simulink library "inp"  (R2021b)
settings: Solver=VariableStepAuto  StartTime=0.0  StopTime=10.0  RelTol=1e-3
undefined symbols (not defined in the file): C_TASK_5MS_S, FALSE, KINP_AcoreReadyToSlp_flg_ovrdflg, KINP_AcoreReadyToSlp_flg_ovrdval, KINP_AllowMovThd_OTA_enum_ovrdflg, KINP_AllowMovThd_OTA_enum_ovrdval, KINP_APSAngleTarget_Deg_ovrdflg, KINP_APSAngleTarget_Deg_ovrdval, KINP_APSDecReq_mps2_ovrdflg, KINP_APSDecReq_mps2_ovrdval, KINP_APSDecReqA_flg_ovrdflg, KINP_APSDecReqA_flg_ovrdval, KINP_APSDFLL_cm_ovrdflg, KINP_APSDFLL_cm_ovrdval, KINP_APSDFLR_cm_ovrdflg, KINP_APSDFLR_cm_ovrdval, KINP_APSDRLL_cm_ovrdflg, KINP_APSDRLL_cm_ovrdval, KINP_APSDRLR_cm_ovrdflg, KINP_APSDRLR_cm_ovrdval, KINP_APSExitCondition_enum_ovrdflg, KINP_APSExitCondition_enum_ovrdval, KINP_APSHWVer_enum_ovrdflg, KINP_APSHWVer_enum_ovrdval, KINP_APSProgressPCT_pct_ovrdflg, KINP_APSProgressPCT_pct_ovrdval, KINP_APSReq_enum_ovrdflg, KINP_APSReq_enum_ovrdval, KINP_APSRQDisplay_enum_ovrdflg, KINP_APSRQDisplay_enum_ovrdval, KINP_APSRqEPASCtrl_flg_ovrdflg, KINP_APSRqEPASCtrl_flg_ovrdval, KINP_APSShiftPosnReq_enum_ovrdval, KINP_APSShiftPosnReq_enum_ovrflg, KINP_APSSpeedCMD_kph_ovrdval, KINP_APSSpeedCMD_kph_ovrflg, KINP_APSStaSystem_enum_ovrdflg, KINP_APSStaSystem_enum_ovrdval, KINP_APSSWVer_enum_ovrdflg, KINP_APSSWVer_enum_ovrdval, KINP_APSVMCReqA_flg_ovrdval, KINP_APSVMCReqA_flg_ovrflg, KINP_APSVRqEPASCtrl_flg_ovrdflg, KINP_APSVRqEPASCtrl_flg_ovrdval, KINP_AuxBattVolmV_mV_ovrdflg, KINP_AuxBattVolmV_mV_ovrdval, KINP_CAASSta_enum_ovrdflg, KINP_CAASSta_enum_ovrdval, KINP_CAASVMCReqA_flg_ovrdval, KINP_CAASVMCReqA_flg_ovrflg, KINP_Chime_enum_ovrdflg, KINP_Chime_enum_ovrdval, KINP_ClearDTCcmd_flg_ovrdflg, KINP_ClearDTCcmd_flg_ovrdval, KINP_EvccAplusPwrUpReq_flg_ovrdflg, KINP_EvccAplusPwrUpReq_flg_ovrdval, KINP_LFID_raw_ovrdval, KINP_LFID_raw_ovrflg, KINP_LRID_raw_ovrdval, KINP_MemOffsetAccX_raw16_ovrdflg ... (+118)
libraries: FVT_lib x942, hcu_lib x1
(part 9 of 31)

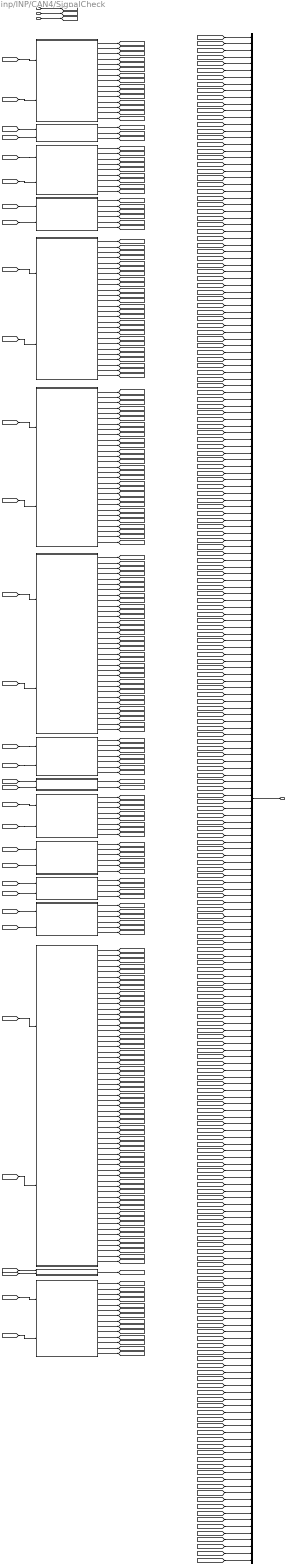
== system inp/INP/CAN4/SignalCheck ==
  inp_CanValid_bus : Inport
  TASK_TIME_S : Inport  Port=2
  BHAL_outputs : Inport  Port=3
  DKC1 : Subsystem
  DKC2 : Subsystem
  PTG1 : Subsystem
  ZONE_DR1 : Subsystem
  ZONE_DR_VCU : Subsystem
  ZONE_FR1 : Subsystem
  ZONE_FR_VCU : Subsystem
  ZONE_L1 : Subsystem
  ZONE_L2 : Subsystem
  ZONE_R1 : Subsystem
  ZONE_R2 : Subsystem
  bus_creator : BusCreator  Inputs=228
  zGW_APTC1 : Subsystem
  zGW_CANFr1 : Subsystem
  zGW_LINDr1 : Subsystem
  zGW_LINFr1 : Subsystem
  zGW_SEAT1 : Subsystem
  inp_Hal_bus : Outport
  wires:
  inp_CanValid_bus/1 -> [inp_CanValid_bus]
  TASK_TIME_S/1 -> [TASK_TIME_S]
  BHAL_outputs/1 -> [BHAL_outputs]
  [BHAL_outputs] -> DKC1/1(BHAL_outputs)
  [inp_CanValid_bus] -> DKC1/2(inp_CanValid_bus)
  DKC1/1(VINP_DKCKeyNumSta_enum) -> [VINP_DKCKeyNumSta_enum]
  DKC1/2(VINP_DKCKeyTypeSta_enum) -> [VINP_DKCKeyTypeSta_enum]
  DKC1/3(VINP_DKCPDkeyAreaRAPSSta_enum) -> [VINP_DKCPDkeyAreaRAPSSta_enum]
  DKC1/4(VINP_DKCParkingModeCmd_enum) -> [VINP_DKCParkingModeCmd_enum]
  DKC1/5(VINP_DKCReVehData_enum) -> [VINP_DKCReVehData_enum]
  DKC1/6(VINP_PCommandToBCM_enum) -> [VINP_PCommandToBCM_enum]
  DKC1/7(VINP_PCommandToPTG_enum) -> [VINP_PCommandToPTG_enum]
  DKC1/8(VINP_PDKeyAreaLockUnlock_enum) -> [VINP_PDKeyAreaLockUnlock_enum]
  DKC1/9(VINP_PDKeyAreaPS_enum) -> [VINP_PDKeyAreaPS_enum]
  DKC1/10(VINP_PDKeyAreaPTG_enum) -> [VINP_PDKeyAreaPTG_enum]
  DKC1/11(VINP_PDKeyWelcome_enum) -> [VINP_PDKeyWelcome_enum]
  DKC1/12(VINP_PDkeyShowIVI_enum) -> [VINP_PDkeyShowIVI_enum]
  DKC1/13(VINP_PKeyMiss_flg) -> [VINP_PKeyMiss_flg]
  DKC1/14(VINP_PKeyMode_enum) -> [VINP_PKeyMode_enum]
  DKC1/15(VINP_PUIDLowPower_flg) -> [VINP_PUIDLowPower_flg]
  [BHAL_outputs] -> DKC2/1(BHAL_outputs)
  [inp_CanValid_bus] -> DKC2/2(inp_CanValid_bus)
  DKC2/1(VINP_EncryptionDATA063_enum) -> [VINP_EncryptionDATA063_enum]
  DKC2/2(VINP_EncryptionDATA64127_enum) -> [VINP_EncryptionDATA64127_enum]
  DKC2/3(VINP_RandomNumberX_enum) -> [VINP_RandomNumberX_enum]
  [BHAL_outputs] -> PTG1/1(BHAL_outputs)
  [inp_CanValid_bus] -> PTG1/2(inp_CanValid_bus)
  PTG1/1(VINP_PTGActiveSta_enum) -> [VINP_PTGActiveSta_enum]
  PTG1/2(VINP_PTGAutoStaus_flg) -> [VINP_PTGAutoStaus_flg]
  PTG1/3(VINP_PTGExist_flg) -> [VINP_PTGExist_flg]
  PTG1/4(VINP_PTGHWVer_enum) -> [VINP_PTGHWVer_enum]
  PTG1/5(VINP_PTGInnerSW2_enum) -> [VINP_PTGInnerSW2_enum]
  PTG1/6(VINP_PTGIsSetHeight_flg) -> [VINP_PTGIsSetHeight_flg]
  PTG1/7(VINP_PTGRDILSta_enum) -> [VINP_PTGRDILSta_enum]
  PTG1/8(VINP_PTGSWVer_enum) -> [VINP_PTGSWVer_enum]
  PTG1/9(VINP_PTGSysSta_enum) -> [VINP_PTGSysSta_enum]
  [BHAL_outputs] -> ZONE_DR1/1(BHAL_outputs)
  [inp_CanValid_bus] -> ZONE_DR1/2(inp_CanValid_bus)
  ZONE_DR1/1(VINP_DrLockSta_flg) -> [VINP_DrLockSta_flg]
  ZONE_DR1/2(VINP_MIRRORFOLDSW_flg) -> [VINP_MIRRORFOLDSW_flg]
  ZONE_DR1/3(VINP_RLTurnLampC_mA) -> [VINP_RLTurnLampC_mA]
  ZONE_DR1/4(VINP_RRTurnLampC_mA) -> [VINP_RRTurnLampC_mA]
  ZONE_DR1/5(VINP_RWiperAS_flg) -> [VINP_RWiperAS_flg]
  ZONE_DR1/6(VINP_RWiperProtection_flg) -> [VINP_RWiperProtection_flg]
  [BHAL_outputs] -> ZONE_DR_VCU/1(BHAL_outputs)
  [inp_CanValid_bus] -> ZONE_DR_VCU/2(inp_CanValid_bus)
  ZONE_DR_VCU/1(VINP_BlowerErr_enum) -> [VINP_BlowerErr_enum]
  ZONE_DR_VCU/2(VINP_DrPMMLVOutPErrLmp_flg) -> [VINP_DrPMMLVOutPErrLmp_flg]
  ZONE_DR_VCU/3(VINP_DrPMMSysErrLmp_flg) -> [VINP_DrPMMSysErrLmp_flg]
  ZONE_DR_VCU/4(VINP_DrSCPSysErrLmp_flg) -> [VINP_DrSCPSysErrLmp_flg]
  ZONE_DR_VCU/5(VINP_DrStdAErrSta_flg) -> [VINP_DrStdAErrSta_flg]
  ZONE_DR_VCU/6(VINP_SolarL_W) -> [VINP_SolarL_W]
  ZONE_DR_VCU/7(VINP_SolarLErr_enum) -> [VINP_SolarLErr_enum]
  ZONE_DR_VCU/8(VINP_SolarR_W) -> [VINP_SolarR_W]
  ZONE_DR_VCU/9(VINP_SolarRErr_enum) -> [VINP_SolarRErr_enum]
  ZONE_DR_VCU/10(VINP_TFaceL_C) -> [VINP_TFaceL_C]
  ZONE_DR_VCU/11(VINP_TFaceLErr_enum) -> [VINP_TFaceLErr_enum]
  ZONE_DR_VCU/12(VINP_TFaceR_C) -> [VINP_TFaceR_C]
  ZONE_DR_VCU/13(VINP_TFaceRErr_enum) -> [VINP_TFaceRErr_enum]
  ZONE_DR_VCU/14(VINP_TFaceRr_C) -> [VINP_TFaceRr_C]
  ZONE_DR_VCU/15(VINP_TFaceRrErr_enum) -> [VINP_TFaceRrErr_enum]
  ZONE_DR_VCU/16(VINP_TFootL_C) -> [VINP_TFootL_C]
  ZONE_DR_VCU/17(VINP_TFootLErr_enum) -> [VINP_TFootLErr_enum]
  ZONE_DR_VCU/18(VINP_TFootR_C) -> [VINP_TFootR_C]
  ZONE_DR_VCU/19(VINP_TFootRErr_enum) -> [VINP_TFootRErr_enum]
  ZONE_DR_VCU/20(VINP_TFootRr_C) -> [VINP_TFootRr_C]
  ZONE_DR_VCU/21(VINP_TFootRrErr_enum) -> [VINP_TFootRrErr_enum]
  ZONE_DR_VCU/22(VINP_Tevap_C) -> [VINP_Tevap_C]
  ZONE_DR_VCU/23(VINP_TevapErr_enum) -> [VINP_TevapErr_enum]
  ZONE_DR_VCU/24(VINP_Tincar_C) -> [VINP_Tincar_C]
  ZONE_DR_VCU/25(VINP_TincarErr_enum) -> [VINP_TincarErr_enum]
  ZONE_DR_VCU/26(VINP_ZoneDrMalfunLevel_enum) -> [VINP_ZoneDrMalfunLevel_enum]
  [BHAL_outputs] -> ZONE_FR1/1(BHAL_outputs)
  [inp_CanValid_bus] -> ZONE_FR1/2(inp_CanValid_bus)
  ZONE_FR1/1(VINP_ChargeInletLockSta_flg) -> [VINP_ChargeInletLockSta_flg]
  ZONE_FR1/2(VINP_CompProEN_flg) -> [VINP_CompProEN_flg]
  ZONE_FR1/3(VINP_FLTurnLampC_mA) -> [VINP_FLTurnLampC_mA]
  ZONE_FR1/4(VINP_FLTurnLightWarning_flg) -> [VINP_FLTurnLightWarning_flg]
  ZONE_FR1/5(VINP_FRTurnLampC_mA) -> [VINP_FRTurnLampC_mA]
  ZONE_FR1/6(VINP_FRTurnLightWarning_flg) -> [VINP_FRTurnLightWarning_flg]
  ZONE_FR1/7(VINP_FWiperAS_flg) -> [VINP_FWiperAS_flg]
  ZONE_FR1/8(VINP_FWiperProtection_flg) -> [VINP_FWiperProtection_flg]
  ZONE_FR1/9(VINP_LADBHibeamIndication_flg) -> [VINP_LADBHibeamIndication_flg]
  ZONE_FR1/10(VINP_LADBOperationStatus_flg) -> [VINP_LADBOperationStatus_flg]
  ZONE_FR1/11(VINP_LADBWarning_flg) -> [VINP_LADBWarning_flg]
  ZONE_FR1/12(VINP_LAHBWarning_flg) -> [VINP_LAHBWarning_flg]
  ZONE_FR1/13(VINP_LDRLWarning_flg) -> [VINP_LDRLWarning_flg]
  ZONE_FR1/14(VINP_LLBWarning_flg) -> [VINP_LLBWarning_flg]
  ZONE_FR1/15(VINP_LpositionLampWarning_flg) -> [VINP_LpositionLampWarning_flg]
  ZONE_FR1/16(VINP_RADBHibeamIndication_flg) -> [VINP_RADBHibeamIndication_flg]
  ZONE_FR1/17(VINP_RADBOperationStatus_flg) -> [VINP_RADBOperationStatus_flg]
  ZONE_FR1/18(VINP_RADBWarning_flg) -> [VINP_RADBWarning_flg]
  ZONE_FR1/19(VINP_RAHBWarning_flg) -> [VINP_RAHBWarning_flg]
  ZONE_FR1/20(VINP_RDRLWarning_flg) -> [VINP_RDRLWarning_flg]
  ZONE_FR1/21(VINP_RLBWarning_flg) -> [VINP_RLBWarning_flg]
  ZONE_FR1/22(VINP_RpositionLampWarning_flg) -> [VINP_RpositionLampWarning_flg]
  ZONE_FR1/23(VINP_TrailerCheck_flg) -> [VINP_TrailerCheck_flg]
  ZONE_FR1/24(VINP_TrailerModeSta_enum) -> [VINP_TrailerModeSta_enum]
  ZONE_FR1/25(VINP_ZFRBCMChargerDoorSWSta_flg) -> [VINP_ZFRBCMChargerDoorSWSta_flg]
  ZONE_FR1/26(VINP_ZFRTHCMCLEVentActYSta_pct) -> [VINP_ZFRTHCMCLEVentActYSta_pct]
  ZONE_FR1/27(VINP_ZFRTHCMCREVentActYSta_pct) -> [VINP_ZFRTHCMCREVentActYSta_pct]
  ZONE_FR1/28(VINP_ZFRTHCMDrEVentActYSta_pct) -> [VINP_ZFRTHCMDrEVentActYSta_pct]
  ZONE_FR1/29(VINP_ZFRTHCMPsEVentActYSta_pct) -> [VINP_ZFRTHCMPsEVentActYSta_pct]
  [BHAL_outputs] -> ZONE_FR_VCU/1(BHAL_outputs)
  [inp_CanValid_bus] -> ZONE_FR_VCU/2(inp_CanValid_bus)
  ZONE_FR_VCU/1(VINP_AGSErr_enum) -> [VINP_AGSErr_enum]
  ZONE_FR_VCU/2(VINP_BatInTemp_C) -> [VINP_BatInTemp_C]
  ZONE_FR_VCU/3(VINP_BatInTempErr_enum) -> [VINP_BatInTempErr_enum]
  ZONE_FR_VCU/4(VINP_BatOutTemp_C) -> [VINP_BatOutTemp_C]
  ZONE_FR_VCU/5(VINP_COMPErr_enum) -> [VINP_COMPErr_enum]
  ZONE_FR_VCU/6(VINP_EACProtectEnable_enum) -> [VINP_EACProtectEnable_enum]
  ZONE_FR_VCU/7(VINP_EWP3Err_enum) -> [VINP_EWP3Err_enum]
  ZONE_FR_VCU/8(VINP_EXV1Err_enum) -> [VINP_EXV1Err_enum]
  ZONE_FR_VCU/9(VINP_EXV2Err_enum) -> [VINP_EXV2Err_enum]
  ZONE_FR_VCU/10(VINP_FanErr_enum) -> [VINP_FanErr_enum]
  ZONE_FR_VCU/11(VINP_FrPMMLimpHomeActReq_flg) -> [VINP_FrPMMLimpHomeActReq_flg]
  ZONE_FR_VCU/12(VINP_MotorInTemp_C) -> [VINP_MotorInTemp_C]
  ZONE_FR_VCU/13(VINP_MotorInTempErr_enum) -> [VINP_MotorInTempErr_enum]
  ZONE_FR_VCU/14(VINP_MotorOutTemp_C) -> [VINP_MotorOutTemp_C]
  ZONE_FR_VCU/15(VINP_MotorOutTempErr_enum) -> [VINP_MotorOutTempErr_enum]
  ZONE_FR_VCU/16(VINP_PTHighP_KPa) -> [VINP_PTHighP_KPa]
  ZONE_FR_VCU/17(VINP_PTHighPErr_enum) -> [VINP_PTHighPErr_enum]
  ZONE_FR_VCU/18(VINP_PTHighTact_C) -> [VINP_PTHighTact_C]
  ZONE_FR_VCU/19(VINP_PTHighTactErr_enum) -> [VINP_PTHighTactErr_enum]
  ZONE_FR_VCU/20(VINP_PTLowP1_KPa) -> [VINP_PTLowP1_KPa]
  ZONE_FR_VCU/21(VINP_PTLowP1Err_enum) -> [VINP_PTLowP1Err_enum]
  ZONE_FR_VCU/22(VINP_PTLowP2_KPa) -> [VINP_PTLowP2_KPa]
  ZONE_FR_VCU/23(VINP_PTLowP2Err_enum) -> [VINP_PTLowP2Err_enum]
  ZONE_FR_VCU/24(VINP_PTLowT1_C) -> [VINP_PTLowT1_C]
  ZONE_FR_VCU/25(VINP_PTLowT1Err_enum) -> [VINP_PTLowT1Err_enum]
  ZONE_FR_VCU/26(VINP_PTLowT2_C) -> [VINP_PTLowT2_C]
  ZONE_FR_VCU/27(VINP_PTLowT2Err_enum) -> [VINP_PTLowT2Err_enum]
  ZONE_FR_VCU/28(VINP_SOTXVErr_enum) -> [VINP_SOTXVErr_enum]
  ZONE_FR_VCU/29(VINP_SOV1Err_enum) -> [VINP_SOV1Err_enum]
  ZONE_FR_VCU/30(VINP_SOV2Err_enum) -> [VINP_SOV2Err_enum]
  ZONE_FR_VCU/31(VINP_SOV3Err_enum) -> [VINP_SOV3Err_enum]
  ZONE_FR_VCU/32(VINP_Tamb_C) -> [VINP_Tamb_C]
  ZONE_FR_VCU/33(VINP_TambErr_enum) -> [VINP_TambErr_enum]
  [BHAL_outputs] -> ZONE_L1/1(BHAL_outputs)
  [inp_CanValid_bus] -> ZONE_L1/2(inp_CanValid_bus)
  ZONE_L1/1(VINP_ZLDSEATAntiSta_flg) -> [VINP_ZLDSEATAntiSta_flg]
  ZONE_L1/2(VINP_ZLDSEATEntryFunSta_flg) -> [VINP_ZLDSEATEntryFunSta_flg]
  ZONE_L1/3(VINP_ZLDSEATErrorSta_flg) -> [VINP_ZLDSEATErrorSta_flg]
  ZONE_L1/4(VINP_ZLDSEATMemSetSta_enum) -> [VINP_ZLDSEATMemSetSta_enum]
  ZONE_L1/5(VINP_ZLDSEATModeSta_enum) -> [VINP_ZLDSEATModeSta_enum]
  ZONE_L1/6(VINP_ZLDSEATVentSta_enum) -> [VINP_ZLDSEATVentSta_enum]
  ZONE_L1/7(VINP_ZLDSEATheaterSta_enum) -> [VINP_ZLDSEATheaterSta_enum]
  [BHAL_outputs] -> ZONE_L2/1(BHAL_outputs)
  [inp_CanValid_bus] -> ZONE_L2/2(inp_CanValid_bus)
  ZONE_L2/1(VINP_ZLAPMWinLFOpenedSta_pct) -> [VINP_ZLAPMWinLFOpenedSta_pct]
  ZONE_L2/2(VINP_ZLAPMWinLROpenedSta_pct) -> [VINP_ZLAPMWinLROpenedSta_pct]
  [BHAL_outputs] -> ZONE_R1/1(BHAL_outputs)
  [inp_CanValid_bus] -> ZONE_R1/2(inp_CanValid_bus)
  ZONE_R1/1(VINP_ZRPSEATErrorSta_flg) -> [VINP_ZRPSEATErrorSta_flg]
  ZONE_R1/2(VINP_ZRPSEATModeSta_enum) -> [VINP_ZRPSEATModeSta_enum]
  ZONE_R1/3(VINP_ZRPSEATVentSta_enum) -> [VINP_ZRPSEATVentSta_enum]
  ZONE_R1/4(VINP_ZRPSEATheaterSta_enum) -> [VINP_ZRPSEATheaterSta_enum]
  ZONE_R1/5(VINP_ZRPTGActiveSta_enum) -> [VINP_ZRPTGActiveSta_enum]
  ZONE_R1/6(VINP_ZRPTGExistSta_flg) -> [VINP_ZRPTGExistSta_flg]
  ZONE_R1/7(VINP_ZRPTGIsSetHeightSta_flg) -> [VINP_ZRPTGIsSetHeightSta_flg]
  ZONE_R1/8(VINP_ZRPTGSysSta_enum) -> [VINP_ZRPTGSysSta_enum]
  [BHAL_outputs] -> ZONE_R2/1(BHAL_outputs)
  [inp_CanValid_bus] -> ZONE_R2/2(inp_CanValid_bus)
  ZONE_R2/1(VINP_ZRAPMWinRFOpenedSta_pct) -> [VINP_ZRAPMWinRFOpenedSta_pct]
  ZONE_R2/2(VINP_ZRAPMWinRROpenedSta_pct) -> [VINP_ZRAPMWinRROpenedSta_pct]
  ZONE_R2/3(VINP_ZRSEATLVentSta_enum) -> [VINP_ZRSEATLVentSta_enum]
  ZONE_R2/4(VINP_ZRSEATMLVentSta_enum) -> [VINP_ZRSEATMLVentSta_enum]
  ZONE_R2/5(VINP_ZRSEATMRVentSta_enum) -> [VINP_ZRSEATMRVentSta_enum]
  ZONE_R2/6(VINP_ZRSEATRVentSta_enum) -> [VINP_ZRSEATRVentSta_enum]
  [BHAL_outputs] -> zGW_APTC1/1(BHAL_outputs)
  [inp_CanValid_bus] -> zGW_APTC1/2(inp_CanValid_bus)
  zGW_APTC1/1(VINP_FrntPTCLeActHeatPwr_W) -> [VINP_FrntPTCLeActHeatPwr_W]
  zGW_APTC1/2(VINP_FrntPTCRearLeActHeatPwr_W) -> [VINP_FrntPTCRearLeActHeatPwr_W]
  zGW_APTC1/3(VINP_FrntPTCRearRiActHeatPwr_W) -> [VINP_FrntPTCRearRiActHeatPwr_W]
  zGW_APTC1/4(VINP_FrntPTCRiActHeatPwr_W) -> [VINP_FrntPTCRiActHeatPwr_W]
  [BHAL_outputs] -> zGW_CANFr1/1(BHAL_outputs)
  [inp_CanValid_bus] -> zGW_CANFr1/2(inp_CanValid_bus)
  zGW_CANFr1/1(VINP_COMPActualPwr_W) -> [VINP_COMPActualPwr_W]
  zGW_CANFr1/2(VINP_COMPConCur_A) -> [VINP_COMPConCur_A]
  zGW_CANFr1/3(VINP_COMPConVolt_V) -> [VINP_COMPConVolt_V]
  zGW_CANFr1/4(VINP_COMPStatorSpd_rpm) -> [VINP_COMPStatorSpd_rpm]
  zGW_CANFr1/5(VINP_PTC1PowerConsumption_kW) -> [VINP_PTC1PowerConsumption_kW]
  zGW_CANFr1/6(VINP_PTCActuPwrHSC6_enum) -> [VINP_PTCActuPwrHSC6_enum]
  [BHAL_outputs] -> zGW_LINDr1/1(BHAL_outputs)
  [inp_CanValid_bus] -> zGW_LINDr1/2(inp_CanValid_bus)
  zGW_LINDr1/1(VINP_CSWDimSw_flg) -> [VINP_CSWDimSw_flg]
  zGW_LINDr1/2(VINP_CSWFWasSwSta_enum) -> [VINP_CSWFWasSwSta_enum]
  zGW_LINDr1/3(VINP_CSWFWipSwSta_enum) -> [VINP_CSWFWipSwSta_enum]
  zGW_LINDr1/4(VINP_CSWPassSWSta_flg) -> [VINP_CSWPassSWSta_flg]
  zGW_LINDr1/5(VINP_CSWRWasSWSta_enum) -> [VINP_CSWRWasSWSta_enum]
  zGW_LINDr1/6(VINP_CSWRWipIntSwSta_enum) -> [VINP_CSWRWipIntSwSta_enum]
  zGW_LINDr1/7(VINP_CSWTurnSwSta_enum) -> [VINP_CSWTurnSwSta_enum]
  zGW_LINDr1/8(VINP_FAPWL01LINResponseError_flg) -> [VINP_FAPWL01LINResponseError_flg]
  zGW_LINDr1/9(VINP_LDrvMotorRelayError_flg) -> [VINP_LDrvMotorRelayError_flg]
  zGW_LINDr1/10(VINP_LDrvMotorRippleError_flg) -> [VINP_LDrvMotorRippleError_flg]
  zGW_LINDr1/11(VINP_LDrvValWdwOpened_pct) -> [VINP_LDrvValWdwOpened_pct]
  zGW_LINDr1/12(VINP_LDrvWdwPositionSts_enum) -> [VINP_LDrvWdwPositionSts_enum]
  zGW_LINDr1/13(VINP_LPasMotorRelayError_flg) -> [VINP_LPasMotorRelayError_flg]
  zGW_LINDr1/14(VINP_LPasMotorRippleError_flg) -> [VINP_LPasMotorRippleError_flg]
  zGW_LINDr1/15(VINP_LPasValWdwOpened_pct) -> [VINP_LPasValWdwOpened_pct]
  zGW_LINDr1/16(VINP_LPasWdwPositionSts_enum) -> [VINP_LPasWdwPositionSts_enum]
  zGW_LINDr1/17(VINP_LRLDMotorRelayError_flg) -> [VINP_LRLDMotorRelayError_flg]
  zGW_LINDr1/18(VINP_LRLDMotorRippleError_flg) -> [VINP_LRLDMotorRippleError_flg]
  zGW_LINDr1/19(VINP_LRLDValWdwOpened_pct) -> [VINP_LRLDValWdwOpened_pct]
  zGW_LINDr1/20(VINP_LRLDWdwPositionSts_enum) -> [VINP_LRLDWdwPositionSts_enum]
  zGW_LINDr1/21(VINP_LRRDMotorRelayError_flg) -> [VINP_LRRDMotorRelayError_flg]
  zGW_LINDr1/22(VINP_LRRDMotorRippleError_flg) -> [VINP_LRRDMotorRippleError_flg]
  zGW_LINDr1/23(VINP_LRRDValWdwOpened_pct) -> [VINP_LRRDValWdwOpened_pct]
  zGW_LINDr1/24(VINP_LRRDWdwPositionSts_enum) -> [VINP_LRRDWdwPositionSts_enum]
  zGW_LINDr1/25(VINP_RAPWL01LINResponseError_flg) -> [VINP_RAPWL01LINResponseError_flg]
  zGW_LINDr1/26(VINP_RLSLampSta_flg) -> [VINP_RLSLampSta_flg]
  zGW_LINDr1/27(VINP_RLSRainSnrWiperCmd_enum) -> [VINP_RLSRainSnrWiperCmd_enum]
  zGW_LINDr1/28(VINP_SWC2LADASSta_flg) -> [VINP_SWC2LADASSta_flg]
  zGW_LINDr1/29(VINP_SWC2LDriveModeSta_flg) -> [VINP_SWC2LDriveModeSta_flg]
  zGW_LINDr1/30(VINP_SWC2LHomeSta_flg) -> [VINP_SWC2LHomeSta_flg]
  zGW_LINDr1/31(VINP_SWC2LLeftSta_flg) -> [VINP_SWC2LLeftSta_flg]
  zGW_LINDr1/32(VINP_SWC2LRightSta_flg) -> [VINP_SWC2LRightSta_flg]
  zGW_LINDr1/33(VINP_SWC2LScrollDownSta_flg) -> [VINP_SWC2LScrollDownSta_flg]
  zGW_LINDr1/34(VINP_SWC2LScrollPressSta_flg) -> [VINP_SWC2LScrollPressSta_flg]
  zGW_LINDr1/35(VINP_SWC2LScrollUpSta_flg) -> [VINP_SWC2LScrollUpSta_flg]
  zGW_LINDr1/36(VINP_SWC2RCustomizeSta_flg) -> [VINP_SWC2RCustomizeSta_flg]
  zGW_LINDr1/37(VINP_SWC2RLeftSta_flg) -> [VINP_SWC2RLeftSta_flg]
  zGW_LINDr1/38(VINP_SWC2RPageSwitchSta_flg) -> [VINP_SWC2RPageSwitchSta_flg]
  zGW_LINDr1/39(VINP_SWC2RRightSta_flg) -> [VINP_SWC2RRightSta_flg]
  zGW_LINDr1/40(VINP_SWC2RScrollDownSta_flg) -> [VINP_SWC2RScrollDownSta_flg]
  zGW_LINDr1/41(VINP_SWC2RScrollPressSta_flg) -> [VINP_SWC2RScrollPressSta_flg]
  zGW_LINDr1/42(VINP_SWC2RScrollUpSta_flg) -> [VINP_SWC2RScrollUpSta_flg]
  zGW_LINDr1/43(VINP_SWC2RVRSta_flg) -> [VINP_SWC2RVRSta_flg]
  zGW_LINDr1/44(VINP_SWCACCSta_flg) -> [VINP_SWCACCSta_flg]
  zGW_LINDr1/45(VINP_SWCCANCELSta_flg) -> [VINP_SWCCANCELSta_flg]
  zGW_LINDr1/46(VINP_SWCDistanceSta_flg) -> [VINP_SWCDistanceSta_flg]
  zGW_LINDr1/47(VINP_SWCDownSta_flg) -> [VINP_SWCDownSta_flg]
  zGW_LINDr1/48(VINP_SWCLKASta_flg) -> [VINP_SWCLKASta_flg]
  zGW_LINDr1/49(VINP_SWCLeftSta_flg) -> [VINP_SWCLeftSta_flg]
  zGW_LINDr1/50(VINP_SWCRegenDown_flg) -> [VINP_SWCRegenDown_flg]
  zGW_LINDr1/51(VINP_SWCRegenUp_flg) -> [VINP_SWCRegenUp_flg]
  zGW_LINDr1/52(VINP_SWCResUpSta_flg) -> [VINP_SWCResUpSta_flg]
  zGW_LINDr1/53(VINP_SWCRightSta_flg) -> [VINP_SWCRightSta_flg]
  zGW_LINDr1/54(VINP_SWCSetdownSta_flg) -> [VINP_SWCSetdownSta_flg]
  zGW_LINDr1/55(VINP_SWCTripSta_flg) -> [VINP_SWCTripSta_flg]
  zGW_LINDr1/56(VINP_SWCUndefinedSta_flg) -> [VINP_SWCUndefinedSta_flg]
  zGW_LINDr1/57(VINP_SWCUpSta_flg) -> [VINP_SWCUpSta_flg]
  zGW_LINDr1/58(VINP_SWCVRSta_flg) -> [VINP_SWCVRSta_flg]
  zGW_LINDr1/59(VINP_SWCmodeSta_flg) -> [VINP_SWCmodeSta_flg]
  [BHAL_outputs] -> zGW_LINFr1/1(BHAL_outputs)
  [inp_CanValid_bus] -> zGW_LINFr1/2(inp_CanValid_bus)
  zGW_LINFr1/1(VINP_AGSActualPosition_enum) -> [VINP_AGSActualPosition_enum]
  [BHAL_outputs] -> zGW_SEAT1/1(BHAL_outputs)
  [inp_CanValid_bus] -> zGW_SEAT1/2(inp_CanValid_bus)
  zGW_SEAT1/1(VINP_DSEATAntiSta_flg) -> [VINP_DSEATAntiSta_flg]
  zGW_SEAT1/2(VINP_DSEATEntryFunSta_flg) -> [VINP_DSEATEntryFunSta_flg]
  zGW_SEAT1/3(VINP_DSEATErrorSta_flg) -> [VINP_DSEATErrorSta_flg]
  zGW_SEAT1/4(VINP_DSEATHWVer_enum) -> [VINP_DSEATHWVer_enum]
  zGW_SEAT1/5(VINP_DSEATMode_enum) -> [VINP_DSEATMode_enum]
  zGW_SEAT1/6(VINP_DSEATSWVer_enum) -> [VINP_DSEATSWVer_enum]
  zGW_SEAT1/7(VINP_DSEATVentSta_enum) -> [VINP_DSEATVentSta_enum]
  zGW_SEAT1/8(VINP_DSEATheatersta_enum) -> [VINP_DSEATheatersta_enum]
  zGW_SEAT1/9(VINP_PSEATErrorSta_flg) -> [VINP_PSEATErrorSta_flg]
  zGW_SEAT1/10(VINP_PSEATHWVer_enum) -> [VINP_PSEATHWVer_enum]
  zGW_SEAT1/11(VINP_PSEATMode_enum) -> [VINP_PSEATMode_enum]
  zGW_SEAT1/12(VINP_PSEATSWVer_enum) -> [VINP_PSEATSWVer_enum]
  zGW_SEAT1/13(VINP_PSEATVentSta_enum) -> [VINP_PSEATVentSta_enum]
  zGW_SEAT1/14(VINP_PSEATheatersta_enum) -> [VINP_PSEATheatersta_enum]
  bus_creator/1 -> inp_Hal_bus/1
  [VINP_DKCKeyNumSta_enum] -> bus_creator/1
  [VINP_DKCKeyTypeSta_enum] -> bus_creator/2
  [VINP_DKCPDkeyAreaRAPSSta_enum] -> bus_creator/3
  [VINP_DKCParkingModeCmd_enum] -> bus_creator/4
  [VINP_DKCReVehData_enum] -> bus_creator/5
  [VINP_PCommandToBCM_enum] -> bus_creator/6
  [VINP_PCommandToPTG_enum] -> bus_creator/7
  [VINP_PDKeyAreaLockUnlock_enum] -> bus_creator/8
  [VINP_PDKeyAreaPS_enum] -> bus_creator/9
  [VINP_PDKeyAreaPTG_enum] -> bus_creator/10
  [VINP_PDKeyWelcome_enum] -> bus_creator/11
  [VINP_PDkeyShowIVI_enum] -> bus_creator/12
  [VINP_PKeyMiss_flg] -> bus_creator/13
  [VINP_PKeyMode_enum] -> bus_creator/14
  [VINP_PUIDLowPower_flg] -> bus_creator/15
  [VINP_EncryptionDATA063_enum] -> bus_creator/16
  [VINP_EncryptionDATA64127_enum] -> bus_creator/17
  [VINP_RandomNumberX_enum] -> bus_creator/18
  [VINP_PTGActiveSta_enum] -> bus_creator/19
  [VINP_PTGAutoStaus_flg] -> bus_creator/20
  [VINP_PTGExist_flg] -> bus_creator/21
  [VINP_PTGHWVer_enum] -> bus_creator/22
  [VINP_PTGInnerSW2_enum] -> bus_creator/23
  [VINP_PTGIsSetHeight_flg] -> bus_creator/24
  [VINP_PTGRDILSta_enum] -> bus_creator/25
  [VINP_PTGSWVer_enum] -> bus_creator/26
  [VINP_PTGSysSta_enum] -> bus_creator/27
  [VINP_DrLockSta_flg] -> bus_creator/28
  [VINP_MIRRORFOLDSW_flg] -> bus_creator/29
  [VINP_RLTurnLampC_mA] -> bus_creator/30
  [VINP_RRTurnLampC_mA] -> bus_creator/31
  [VINP_RWiperAS_flg] -> bus_creator/32
  [VINP_RWiperProtection_flg] -> bus_creator/33
  [VINP_BlowerErr_enum] -> bus_creator/34
  [VINP_DrPMMLVOutPErrLmp_flg] -> bus_creator/35
  [VINP_DrPMMSysErrLmp_flg] -> bus_creator/36
  [VINP_DrSCPSysErrLmp_flg] -> bus_creator/37
  [VINP_DrStdAErrSta_flg] -> bus_creator/38
  [VINP_SolarL_W] -> bus_creator/39
  [VINP_SolarLErr_enum] -> bus_creator/40
  [VINP_SolarR_W] -> bus_creator/41
  [VINP_SolarRErr_enum] -> bus_creator/42
  [VINP_TFaceL_C] -> bus_creator/43
  [VINP_TFaceLErr_enum] -> bus_creator/44
  [VINP_TFaceR_C] -> bus_creator/45
  [VINP_TFaceRErr_enum] -> bus_creator/46
  [VINP_TFaceRr_C] -> bus_creator/47
  [VINP_TFaceRrErr_enum] -> bus_creator/48
  [VINP_TFootL_C] -> bus_creator/49
  [VINP_TFootLErr_enum] -> bus_creator/50
  [VINP_TFootR_C] -> bus_creator/51
  [VINP_TFootRErr_enum] -> bus_creator/52
  [VINP_TFootRr_C] -> bus_creator/53
  [VINP_TFootRrErr_enum] -> bus_creator/54
  [VINP_Tevap_C] -> bus_creator/55
  [VINP_TevapErr_enum] -> bus_creator/56
  [VINP_Tincar_C] -> bus_creator/57
  [VINP_TincarErr_enum] -> bus_creator/58
  [VINP_ZoneDrMalfunLevel_enum] -> bus_creator/59
  [VINP_ChargeInletLockSta_flg] -> bus_creator/60
  [VINP_CompProEN_flg] -> bus_creator/61
  [VINP_FLTurnLampC_mA] -> bus_creator/62
  [VINP_FLTurnLightWarning_flg] -> bus_creator/63
  [VINP_FRTurnLampC_mA] -> bus_creator/64
  [VINP_FRTurnLightWarning_flg] -> bus_creator/65
  [VINP_FWiperAS_flg] -> bus_creator/66
  [VINP_FWiperProtection_flg] -> bus_creator/67
  [VINP_LADBHibeamIndication_flg] -> bus_creator/68
  [VINP_LADBOperationStatus_flg] -> bus_creator/69
  [VINP_LADBWarning_flg] -> bus_creator/70
  [VINP_LAHBWarning_flg] -> bus_creator/71
  [VINP_LDRLWarning_flg] -> bus_creator/72
  [VINP_LLBWarning_flg] -> bus_creator/73
  [VINP_LpositionLampWarning_flg] -> bus_creator/74
  [VINP_RADBHibeamIndication_flg] -> bus_creator/75
  [VINP_RADBOperationStatus_flg] -> bus_creator/76
  [VINP_RADBWarning_flg] -> bus_creator/77
  [VINP_RAHBWarning_flg] -> bus_creator/78
  [VINP_RDRLWarning_flg] -> bus_creator/79
  [VINP_RLBWarning_flg] -> bus_creator/80
  [VINP_RpositionLampWarning_flg] -> bus_creator/81
  [VINP_TrailerCheck_flg] -> bus_creator/82
  [VINP_TrailerModeSta_enum] -> bus_creator/83
  [VINP_ZFRBCMChargerDoorSWSta_flg] -> bus_creator/84
  [VINP_ZFRTHCMCLEVentActYSta_pct] -> bus_creator/85
  [VINP_ZFRTHCMCREVentActYSta_pct] -> bus_creator/86
  [VINP_ZFRTHCMDrEVentActYSta_pct] -> bus_creator/87
  [VINP_ZFRTHCMPsEVentActYSta_pct] -> bus_creator/88
  [VINP_AGSErr_enum] -> bus_creator/89
  [VINP_BatInTemp_C] -> bus_creator/90
  [VINP_BatInTempErr_enum] -> bus_creator/91
  [VINP_BatOutTemp_C] -> bus_creator/92
  [VINP_COMPErr_enum] -> bus_creator/93
  [VINP_EACProtectEnable_enum] -> bus_creator/94
  [VINP_EWP3Err_enum] -> bus_creator/95
  [VINP_EXV1Err_enum] -> bus_creator/96
  [VINP_EXV2Err_enum] -> bus_creator/97
  [VINP_FanErr_enum] -> bus_creator/98
  [VINP_FrPMMLimpHomeActReq_flg] -> bus_creator/99
  [VINP_MotorInTemp_C] -> bus_creator/100
  [VINP_MotorInTempErr_enum] -> bus_creator/101
  [VINP_MotorOutTemp_C] -> bus_creator/102
  [VINP_MotorOutTempErr_enum] -> bus_creator/103
  [VINP_PTHighP_KPa] -> bus_creator/104
  [VINP_PTHighPErr_enum] -> bus_creator/105
  [VINP_PTHighTact_C] -> bus_creator/106
  [VINP_PTHighTactErr_enum] -> bus_creator/107
  [VINP_PTLowP1_KPa] -> bus_creator/108
  [VINP_PTLowP1Err_enum] -> bus_creator/109
  [VINP_PTLowP2_KPa] -> bus_creator/110
  [VINP_PTLowP2Err_enum] -> bus_creator/111
  [VINP_PTLowT1_C] -> bus_creator/112
  [VINP_PTLowT1Err_enum] -> bus_creator/113
  [VINP_PTLowT2_C] -> bus_creator/114
  [VINP_PTLowT2Err_enum] -> bus_creator/115
  [VINP_SOTXVErr_enum] -> bus_creator/116
  [VINP_SOV1Err_enum] -> bus_creator/117
  [VINP_SOV2Err_enum] -> bus_creator/118
  [VINP_SOV3Err_enum] -> bus_creator/119
  [VINP_Tamb_C] -> bus_creator/120
  [VINP_TambErr_enum] -> bus_creator/121
  [VINP_ZLDSEATAntiSta_flg] -> bus_creator/122
  [VINP_ZLDSEATEntryFunSta_flg] -> bus_creator/123
  [VINP_ZLDSEATErrorSta_flg] -> bus_creator/124
  [VINP_ZLDSEATMemSetSta_enum] -> bus_creator/125
  [VINP_ZLDSEATModeSta_enum] -> bus_creator/126
  [VINP_ZLDSEATVentSta_enum] -> bus_creator/127
  [VINP_ZLDSEATheaterSta_enum] -> bus_creator/128
  [VINP_ZLAPMWinLFOpenedSta_pct] -> bus_creator/129
  [VINP_ZLAPMWinLROpenedSta_pct] -> bus_creator/130
  [VINP_ZRPSEATErrorSta_flg] -> bus_creator/131
  [VINP_ZRPSEATModeSta_enum] -> bus_creator/132
  [VINP_ZRPSEATVentSta_enum] -> bus_creator/133
  [VINP_ZRPSEATheaterSta_enum] -> bus_creator/134
  [VINP_ZRPTGActiveSta_enum] -> bus_creator/135
  [VINP_ZRPTGExistSta_flg] -> bus_creator/136
  [VINP_ZRPTGIsSetHeightSta_flg] -> bus_creator/137
  [VINP_ZRPTGSysSta_enum] -> bus_creator/138
  [VINP_ZRAPMWinRFOpenedSta_pct] -> bus_creator/139
  [VINP_ZRAPMWinRROpenedSta_pct] -> bus_creator/140
  [VINP_ZRSEATLVentSta_enum] -> bus_creator/141
  [VINP_ZRSEATMLVentSta_enum] -> bus_creator/142
  [VINP_ZRSEATMRVentSta_enum] -> bus_creator/143
  [VINP_ZRSEATRVentSta_enum] -> bus_creator/144
  [VINP_FrntPTCLeActHeatPwr_W] -> bus_creator/145
  [VINP_FrntPTCRearLeActHeatPwr_W] -> bus_creator/146
  [VINP_FrntPTCRearRiActHeatPwr_W] -> bus_creator/147
  [VINP_FrntPTCRiActHeatPwr_W] -> bus_creator/148
  [VINP_COMPActualPwr_W] -> bus_creator/149
  [VINP_COMPConCur_A] -> bus_creator/150
  [VINP_COMPConVolt_V] -> bus_creator/151
  [VINP_COMPStatorSpd_rpm] -> bus_creator/152
  [VINP_PTC1PowerConsumption_kW] -> bus_creator/153
  [VINP_PTCActuPwrHSC6_enum] -> bus_creator/154
  [VINP_CSWDimSw_flg] -> bus_creator/155
  [VINP_CSWFWasSwSta_enum] -> bus_creator/156
  [VINP_CSWFWipSwSta_enum] -> bus_creator/157
  [VINP_CSWPassSWSta_flg] -> bus_creator/158
  [VINP_CSWRWasSWSta_enum] -> bus_creator/159
  [VINP_CSWRWipIntSwSta_enum] -> bus_creator/160
  [VINP_CSWTurnSwSta_enum] -> bus_creator/161
  [VINP_FAPWL01LINResponseError_flg] -> bus_creator/162
  [VINP_LDrvMotorRelayError_flg] -> bus_creator/163
  [VINP_LDrvMotorRippleError_flg] -> bus_creator/164
  [VINP_LDrvValWdwOpened_pct] -> bus_creator/165
  [VINP_LDrvWdwPositionSts_enum] -> bus_creator/166
  [VINP_LPasMotorRelayError_flg] -> bus_creator/167
  [VINP_LPasMotorRippleError_flg] -> bus_creator/168
  [VINP_LPasValWdwOpened_pct] -> bus_creator/169
  [VINP_LPasWdwPositionSts_enum] -> bus_creator/170
  [VINP_LRLDMotorRelayError_flg] -> bus_creator/171
  [VINP_LRLDMotorRippleError_flg] -> bus_creator/172
  [VINP_LRLDValWdwOpened_pct] -> bus_creator/173
  [VINP_LRLDWdwPositionSts_enum] -> bus_creator/174
  [VINP_LRRDMotorRelayError_flg] -> bus_creator/175
  [VINP_LRRDMotorRippleError_flg] -> bus_creator/176
  [VINP_LRRDValWdwOpened_pct] -> bus_creator/177
  [VINP_LRRDWdwPositionSts_enum] -> bus_creator/178
  [VINP_RAPWL01LINResponseError_flg] -> bus_creator/179
  [VINP_RLSLampSta_flg] -> bus_creator/180
  [VINP_RLSRainSnrWiperCmd_enum] -> bus_creator/181
  [VINP_SWC2LADASSta_flg] -> bus_creator/182
  [VINP_SWC2LDriveModeSta_flg] -> bus_creator/183
  [VINP_SWC2LHomeSta_flg] -> bus_creator/184
  [VINP_SWC2LLeftSta_flg] -> bus_creator/185
  [VINP_SWC2LRightSta_flg] -> bus_creator/186
  [VINP_SWC2LScrollDownSta_flg] -> bus_creator/187
  [VINP_SWC2LScrollPressSta_flg] -> bus_creator/188
  [VINP_SWC2LScrollUpSta_flg] -> bus_creator/189
  [VINP_SWC2RCustomizeSta_flg] -> bus_creator/190
  [VINP_SWC2RLeftSta_flg] -> bus_creator/191
  [VINP_SWC2RPageSwitchSta_flg] -> bus_creator/192
  [VINP_SWC2RRightSta_flg] -> bus_creator/193
  [VINP_SWC2RScrollDownSta_flg] -> bus_creator/194
  [VINP_SWC2RScrollPressSta_flg] -> bus_creator/195
  [VINP_SWC2RScrollUpSta_flg] -> bus_creator/196
  [VINP_SWC2RVRSta_flg] -> bus_creator/197
  [VINP_SWCACCSta_flg] -> bus_creator/198
  [VINP_SWCCANCELSta_flg] -> bus_creator/199
  [VINP_SWCDistanceSta_flg] -> bus_creator/200
  [VINP_SWCDownSta_flg] -> bus_creator/201
  [VINP_SWCLKASta_flg] -> bus_creator/202
  [VINP_SWCLeftSta_flg] -> bus_creator/203
  [VINP_SWCRegenDown_flg] -> bus_creator/204
  [VINP_SWCRegenUp_flg] -> bus_creator/205
  [VINP_SWCResUpSta_flg] -> bus_creator/206
  [VINP_SWCRightSta_flg] -> bus_creator/207
  [VINP_SWCSetdownSta_flg] -> bus_creator/208
  [VINP_SWCTripSta_flg] -> bus_creator/209
  [VINP_SWCUndefinedSta_flg] -> bus_creator/210
  [VINP_SWCUpSta_flg] -> bus_creator/211
  [VINP_SWCVRSta_flg] -> bus_creator/212
  [VINP_SWCmodeSta_flg] -> bus_creator/213
  [VINP_AGSActualPosition_enum] -> bus_creator/214
  [VINP_DSEATAntiSta_flg] -> bus_creator/215
  [VINP_DSEATEntryFunSta_flg] -> bus_creator/216
  [VINP_DSEATErrorSta_flg] -> bus_creator/217
  [VINP_DSEATHWVer_enum] -> bus_creator/218
  [VINP_DSEATMode_enum] -> bus_creator/219
  [VINP_DSEATSWVer_enum] -> bus_creator/220
  [VINP_DSEATVentSta_enum] -> bus_creator/221
  [VINP_DSEATheatersta_enum] -> bus_creator/222
  [VINP_PSEATErrorSta_flg] -> bus_creator/223
  [VINP_PSEATHWVer_enum] -> bus_creator/224
  [VINP_PSEATMode_enum] -> bus_creator/225
  [VINP_PSEATSWVer_enum] -> bus_creator/226
  [VINP_PSEATVentSta_enum] -> bus_creator/227
  [VINP_PSEATheatersta_enum] -> bus_creator/228

== system inp/INP/CAN5/CommunicationCheck ==
  BHAL_outputs : Inport
  CANMsgInvalidTBOX1 : FVT_lib/inp/CAN_Msg_Validity_Process_template  SystemSampleTime=-1  VariantActivationTime=update diagram  Latency=0  AutoFrameSizeCalculation=off
      link override ovrdflg: Value=KINP_CANMsgInvalidTBOX1_flg_ovrdflg
      link override ovrdval: Value=KINP_CANMsgInvalidTBOX1_flg_ovrdval
  CANMsgInvalidTBOX2 : FVT_lib/inp/CAN_Msg_Validity_Process_template  SystemSampleTime=-1  VariantActivationTime=update diagram  Latency=0  AutoFrameSizeCalculation=off
      link override ovrdflg: Value=KINP_CANMsgInvalidTBOX2_flg_ovrdflg
      link override ovrdval: Value=KINP_CANMsgInvalidTBOX2_flg_ovrdval
  CANMsgInvalidTBOX3 : FVT_lib/inp/CAN_Msg_Validity_Process_template  SystemSampleTime=-1  VariantActivationTime=update diagram  Latency=0  AutoFrameSizeCalculation=off
      link override ovrdflg: Value=KINP_CANMsgInvalidTBOX3_flg_ovrdflg
      link override ovrdval: Value=KINP_CANMsgInvalidTBOX3_flg_ovrdval
  bus_creator : BusCreator  Inputs=3
  bus_selector : BusSelector  OutputSignals=VHAL_CANMsgInvalidTBOX1_flg,VHAL_CANMsgInvalidTBOX2_flg,VHAL_CANMsgInvalidTBOX3_flg
  not1 : Logic  Operator=NOT  AllPortsSameDT=off  OutDataTypeStr=boolean
  not2 : Logic  Operator=NOT  AllPortsSameDT=off  OutDataTypeStr=boolean
  not3 : Logic  Operator=NOT  AllPortsSameDT=off  OutDataTypeStr=boolean
  inp_CanValid_bus : Outport
  wires:
  BHAL_outputs/1 -> [BHAL_outputs]
  bus_selector/1 -> CANMsgInvalidTBOX1/1  "<VHAL_CANMsgInvalidTBOX1_flg>"
  CANMsgInvalidTBOX1/1 -> not1/1
  not1/1 -> bus_creator/1  "VINP_CANMsgValidTBOX1_flg"
  bus_selector/2 -> CANMsgInvalidTBOX2/1  "<VHAL_CANMsgInvalidTBOX2_flg>"
  CANMsgInvalidTBOX2/1 -> not2/1
  not2/1 -> bus_creator/2  "VINP_CANMsgValidTBOX2_flg"
  bus_selector/3 -> CANMsgInvalidTBOX3/1  "<VHAL_CANMsgInvalidTBOX3_flg>"
  CANMsgInvalidTBOX3/1 -> not3/1
  not3/1 -> bus_creator/3  "VINP_CANMsgValidTBOX3_flg"
  [BHAL_outputs] -> bus_selector/1
  bus_creator/1 -> inp_CanValid_bus/1

== system inp/INP/CAN5/CreateBus ==
  inp_CanValid_bus : Inport
  inp_Hal_bus : Inport  Port=2
  UnitConverter_{1..3,9,11} (5 alike) : DataTypeConversion  OutDataTypeStr=boolean
  UnitConverter_{5,10,15..31} (19 alike) : DataTypeConversion  OutDataTypeStr=single
  UnitConverter_{4,6,8,12..14} (6 alike) : DataTypeConversion  OutDataTypeStr=uint8
  UnitConverter_32 : DataTypeConversion  OutDataTypeStr=uint32
  UnitConverter_33 : DataTypeConversion  OutDataTypeStr=uint32
  UnitConverter_7 : DataTypeConversion  OutDataTypeStr=uint16
  bus_creator : BusCreator  Inputs=33
  bus_selector : BusSelector  OutputSignals=VINP_CANMsgValidTBOX1_flg,VINP_CANMsgValidTBOX2_flg,VINP_CANMsgValidTBOX3_flg
  bus_selector_1 : BusSelector  OutputSignals=VINP_CbnPreACEnaReq_enum,VINP_PowerOffTSet_cnt,VINP_ReOutsideMirror_enum,VINP_ReDoorLock_enum,VINP_RePwrReqTbox_enum,VINP_ReRadio_flg,VINP_RemoteACTemp_C,VINP_RemoteAutoReq_flg,VINP_TBOXNETSIGSTR_enum,VINP_TBOXRemotePW_enum,VINP_TBOXTESTSTATUS_enum,VINP_TimeSyncFromBSDay_DAY,VINP_TimeSyncFromBSHour_hr,VINP_TimeSyncFromBSMinute_min,VINP_TimeSyncFromBSMonth_MONTH,VINP_TimeSyncFromBSSecond_s,VINP_TimeSyncFromBSYear_YEAR,VINP_ChargePercentSet_pct,VINP_ReserveChargeOFFDay_DAY,VINP_ReserveChargeOFFHour_hr,VINP_ReserveChargeOFFMinute_min,VINP_ReserveChargeOFFMonth_MONTH,VINP_ReserveChargeOFFYear_YEAR,VINP_ReserveChargeOnDay_DAY,VINP_ReserveChargeOnHour_hr,VINP_ReserveChargeOnMinute_min,VINP_ReserveChargeOnMonth_MONTH,VINP_ReserveChargeOnYear_YEAR,VINP_TBOXHWVER_enum,VINP_TBOXSWVER_enum
  BINP_outputs : Outport
  wires:
  inp_CanValid_bus/1 -> [inp_CanValid_bus]
  inp_Hal_bus/1 -> [inp_Hal_bus]
  bus_selector/1 -> UnitConverter_1/1  "<VINP_CANMsgValidTBOX1_flg>"
  UnitConverter_1/1 -> bus_creator/1  "VINP_CANMsgValidTBOX1_flg"
  bus_selector/2 -> UnitConverter_2/1  "<VINP_CANMsgValidTBOX2_flg>"
  UnitConverter_2/1 -> bus_creator/2  "VINP_CANMsgValidTBOX2_flg"
  bus_selector/3 -> UnitConverter_3/1  "<VINP_CANMsgValidTBOX3_flg>"
  UnitConverter_3/1 -> bus_creator/3  "VINP_CANMsgValidTBOX3_flg"
  bus_selector_1/1 -> UnitConverter_4/1  "<VINP_CbnPreACEnaReq_enum>"
  UnitConverter_4/1 -> bus_creator/4  "VINP_CbnPreACEnaReq_enum"
  bus_selector_1/2 -> UnitConverter_5/1  "<VINP_PowerOffTSet_cnt>"
  UnitConverter_5/1 -> bus_creator/5  "VINP_PowerOffTSet_cnt"
  bus_selector_1/3 -> UnitConverter_6/1  "<VINP_ReOutsideMirror_enum>"
  UnitConverter_6/1 -> bus_creator/6  "VINP_ReOutsideMirror_enum"
  bus_selector_1/4 -> UnitConverter_7/1  "<VINP_ReDoorLock_enum>"
  UnitConverter_7/1 -> bus_creator/7  "VINP_ReDoorLock_enum"
  bus_selector_1/5 -> UnitConverter_8/1  "<VINP_RePwrReqTbox_enum>"
  UnitConverter_8/1 -> bus_creator/8  "VINP_RePwrReqTbox_enum"
  bus_selector_1/6 -> UnitConverter_9/1  "<VINP_ReRadio_flg>"
  UnitConverter_9/1 -> bus_creator/9  "VINP_ReRadio_flg"
  bus_selector_1/7 -> UnitConverter_10/1  "<VINP_RemoteACTemp_C>"
  UnitConverter_10/1 -> bus_creator/10  "VINP_RemoteACTemp_C"
  bus_selector_1/8 -> UnitConverter_11/1  "<VINP_RemoteAutoReq_flg>"
  UnitConverter_11/1 -> bus_creator/11  "VINP_RemoteAutoReq_flg"
  bus_selector_1/9 -> UnitConverter_12/1  "<VINP_TBOXNETSIGSTR_enum>"
  UnitConverter_12/1 -> bus_creator/12  "VINP_TBOXNETSIGSTR_enum"
  bus_selector_1/10 -> UnitConverter_13/1  "<VINP_TBOXRemotePW_enum>"
  UnitConverter_13/1 -> bus_creator/13  "VINP_TBOXRemotePW_enum"
  bus_selector_1/11 -> UnitConverter_14/1  "<VINP_TBOXTESTSTATUS_enum>"
  UnitConverter_14/1 -> bus_creator/14  "VINP_TBOXTESTSTATUS_enum"
  bus_selector_1/12 -> UnitConverter_15/1  "<VINP_TimeSyncFromBSDay_DAY>"
  UnitConverter_15/1 -> bus_creator/15  "VINP_TimeSyncFromBSDay_DAY"
  bus_selector_1/13 -> UnitConverter_16/1  "<VINP_TimeSyncFromBSHour_hr>"
  UnitConverter_16/1 -> bus_creator/16  "VINP_TimeSyncFromBSHour_hr"
  bus_selector_1/14 -> UnitConverter_17/1  "<VINP_TimeSyncFromBSMinute_min>"
  UnitConverter_17/1 -> bus_creator/17  "VINP_TimeSyncFromBSMinute_min"
  bus_selector_1/15 -> UnitConverter_18/1  "<VINP_TimeSyncFromBSMonth_MONTH>"
  UnitConverter_18/1 -> bus_creator/18  "VINP_TimeSyncFromBSMonth_MONTH"
  bus_selector_1/16 -> UnitConverter_19/1  "<VINP_TimeSyncFromBSSecond_s>"
  UnitConverter_19/1 -> bus_creator/19  "VINP_TimeSyncFromBSSecond_s"
  bus_selector_1/17 -> UnitConverter_20/1  "<VINP_TimeSyncFromBSYear_YEAR>"
  UnitConverter_20/1 -> bus_creator/20  "VINP_TimeSyncFromBSYear_YEAR"
  bus_selector_1/18 -> UnitConverter_21/1  "<VINP_ChargePercentSet_pct>"
  UnitConverter_21/1 -> bus_creator/21  "VINP_ChargePercentSet_pct"
  bus_selector_1/19 -> UnitConverter_22/1  "<VINP_ReserveChargeOFFDay_DAY>"
  UnitConverter_22/1 -> bus_creator/22  "VINP_ReserveChargeOFFDay_DAY"
  bus_selector_1/20 -> UnitConverter_23/1  "<VINP_ReserveChargeOFFHour_hr>"
  UnitConverter_23/1 -> bus_creator/23  "VINP_ReserveChargeOFFHour_hr"
  bus_selector_1/21 -> UnitConverter_24/1  "<VINP_ReserveChargeOFFMinute_min>"
  UnitConverter_24/1 -> bus_creator/24  "VINP_ReserveChargeOFFMinute_min"
  bus_selector_1/22 -> UnitConverter_25/1  "<VINP_ReserveChargeOFFMonth_MONTH>"
  UnitConverter_25/1 -> bus_creator/25  "VINP_ReserveChargeOFFMonth_MONTH"
  bus_selector_1/23 -> UnitConverter_26/1  "<VINP_ReserveChargeOFFYear_YEAR>"
  UnitConverter_26/1 -> bus_creator/26  "VINP_ReserveChargeOFFYear_YEAR"
  bus_selector_1/24 -> UnitConverter_27/1  "<VINP_ReserveChargeOnDay_DAY>"
  UnitConverter_27/1 -> bus_creator/27  "VINP_ReserveChargeOnDay_DAY"
  bus_selector_1/25 -> UnitConverter_28/1  "<VINP_ReserveChargeOnHour_hr>"
  UnitConverter_28/1 -> bus_creator/28  "VINP_ReserveChargeOnHour_hr"
  bus_selector_1/26 -> UnitConverter_29/1  "<VINP_ReserveChargeOnMinute_min>"
  UnitConverter_29/1 -> bus_creator/29  "VINP_ReserveChargeOnMinute_min"
  bus_selector_1/27 -> UnitConverter_30/1  "<VINP_ReserveChargeOnMonth_MONTH>"
  UnitConverter_30/1 -> bus_creator/30  "VINP_ReserveChargeOnMonth_MONTH"
  bus_selector_1/28 -> UnitConverter_31/1  "<VINP_ReserveChargeOnYear_YEAR>"
  UnitConverter_31/1 -> bus_creator/31  "VINP_ReserveChargeOnYear_YEAR"
  bus_selector_1/29 -> UnitConverter_32/1  "<VINP_TBOXHWVER_enum>"
  UnitConverter_32/1 -> bus_creator/32  "VINP_TBOXHWVER_enum"
  bus_selector_1/30 -> UnitConverter_33/1  "<VINP_TBOXSWVER_enum>"
  UnitConverter_33/1 -> bus_creator/33  "VINP_TBOXSWVER_enum"
  [inp_CanValid_bus] -> bus_selector/1
  [inp_Hal_bus] -> bus_selector_1/1
  bus_creator/1 -> BINP_outputs/1

== system inp/INP/CAN5/SignalCheck ==
  inp_CanValid_bus : Inport
  TASK_TIME_S : Inport  Port=2
  BHAL_outputs : Inport  Port=3
  TBOX1 : Subsystem
  TBOX2 : Subsystem
  TBOX3 : Subsystem
  bus_creator : BusCreator  Inputs=30
  inp_Hal_bus : Outport
  wires:
  inp_CanValid_bus/1 -> [inp_CanValid_bus]
  TASK_TIME_S/1 -> [TASK_TIME_S]
  BHAL_outputs/1 -> [BHAL_outputs]
  [BHAL_outputs] -> TBOX1/1(BHAL_outputs)
  [inp_CanValid_bus] -> TBOX1/2(inp_CanValid_bus)
  TBOX1/1(VINP_CbnPreACEnaReq_enum) -> [VINP_CbnPreACEnaReq_enum]
  TBOX1/2(VINP_PowerOffTSet_cnt) -> [VINP_PowerOffTSet_cnt]
  TBOX1/3(VINP_ReOutsideMirror_enum) -> [VINP_ReOutsideMirror_enum]
  TBOX1/4(VINP_ReDoorLock_enum) -> [VINP_ReDoorLock_enum]
  TBOX1/5(VINP_RePwrReqTbox_enum) -> [VINP_RePwrReqTbox_enum]
  TBOX1/6(VINP_ReRadio_flg) -> [VINP_ReRadio_flg]
  TBOX1/7(VINP_RemoteACTemp_C) -> [VINP_RemoteACTemp_C]
  TBOX1/8(VINP_RemoteAutoReq_flg) -> [VINP_RemoteAutoReq_flg]
  TBOX1/9(VINP_TBOXNETSIGSTR_enum) -> [VINP_TBOXNETSIGSTR_enum]
  TBOX1/10(VINP_TBOXRemotePW_enum) -> [VINP_TBOXRemotePW_enum]
  TBOX1/11(VINP_TBOXTESTSTATUS_enum) -> [VINP_TBOXTESTSTATUS_enum]
  [BHAL_outputs] -> TBOX2/1(BHAL_outputs)
  [inp_CanValid_bus] -> TBOX2/2(inp_CanValid_bus)
  TBOX2/1(VINP_TimeSyncFromBSDay_DAY) -> [VINP_TimeSyncFromBSDay_DAY]
  TBOX2/2(VINP_TimeSyncFromBSHour_hr) -> [VINP_TimeSyncFromBSHour_hr]
  TBOX2/3(VINP_TimeSyncFromBSMinute_min) -> [VINP_TimeSyncFromBSMinute_min]
  TBOX2/4(VINP_TimeSyncFromBSMonth_MONTH) -> [VINP_TimeSyncFromBSMonth_MONTH]
  TBOX2/5(VINP_TimeSyncFromBSSecond_s) -> [VINP_TimeSyncFromBSSecond_s]
  TBOX2/6(VINP_TimeSyncFromBSYear_YEAR) -> [VINP_TimeSyncFromBSYear_YEAR]
  [BHAL_outputs] -> TBOX3/1(BHAL_outputs)
  [inp_CanValid_bus] -> TBOX3/2(inp_CanValid_bus)
  TBOX3/1(VINP_ChargePercentSet_pct) -> [VINP_ChargePercentSet_pct]
  TBOX3/2(VINP_ReserveChargeOFFDay_DAY) -> [VINP_ReserveChargeOFFDay_DAY]
  TBOX3/3(VINP_ReserveChargeOFFHour_hr) -> [VINP_ReserveChargeOFFHour_hr]
  TBOX3/4(VINP_ReserveChargeOFFMinute_min) -> [VINP_ReserveChargeOFFMinute_min]
  TBOX3/5(VINP_ReserveChargeOFFMonth_MONTH) -> [VINP_ReserveChargeOFFMonth_MONTH]
  TBOX3/6(VINP_ReserveChargeOFFYear_YEAR) -> [VINP_ReserveChargeOFFYear_YEAR]
  TBOX3/7(VINP_ReserveChargeOnDay_DAY) -> [VINP_ReserveChargeOnDay_DAY]
  TBOX3/8(VINP_ReserveChargeOnHour_hr) -> [VINP_ReserveChargeOnHour_hr]
  TBOX3/9(VINP_ReserveChargeOnMinute_min) -> [VINP_ReserveChargeOnMinute_min]
  TBOX3/10(VINP_ReserveChargeOnMonth_MONTH) -> [VINP_ReserveChargeOnMonth_MONTH]
  TBOX3/11(VINP_ReserveChargeOnYear_YEAR) -> [VINP_ReserveChargeOnYear_YEAR]
  TBOX3/12(VINP_TBOXHWVER_enum) -> [VINP_TBOXHWVER_enum]
  TBOX3/13(VINP_TBOXSWVER_enum) -> [VINP_TBOXSWVER_enum]
  bus_creator/1 -> inp_Hal_bus/1
  [VINP_CbnPreACEnaReq_enum] -> bus_creator/1
  [VINP_PowerOffTSet_cnt] -> bus_creator/2
  [VINP_ReOutsideMirror_enum] -> bus_creator/3
  [VINP_ReDoorLock_enum] -> bus_creator/4
  [VINP_RePwrReqTbox_enum] -> bus_creator/5
  [VINP_ReRadio_flg] -> bus_creator/6
  [VINP_RemoteACTemp_C] -> bus_creator/7
  [VINP_RemoteAutoReq_flg] -> bus_creator/8
  [VINP_TBOXNETSIGSTR_enum] -> bus_creator/9
  [VINP_TBOXRemotePW_enum] -> bus_creator/10
  [VINP_TBOXTESTSTATUS_enum] -> bus_creator/11
  [VINP_TimeSyncFromBSDay_DAY] -> bus_creator/12
  [VINP_TimeSyncFromBSHour_hr] -> bus_creator/13
  [VINP_TimeSyncFromBSMinute_min] -> bus_creator/14
  [VINP_TimeSyncFromBSMonth_MONTH] -> bus_creator/15
  [VINP_TimeSyncFromBSSecond_s] -> bus_creator/16
  [VINP_TimeSyncFromBSYear_YEAR] -> bus_creator/17
  [VINP_ChargePercentSet_pct] -> bus_creator/18
  [VINP_ReserveChargeOFFDay_DAY] -> bus_creator/19
  [VINP_ReserveChargeOFFHour_hr] -> bus_creator/20
  [VINP_ReserveChargeOFFMinute_min] -> bus_creator/21
  [VINP_ReserveChargeOFFMonth_MONTH] -> bus_creator/22
  [VINP_ReserveChargeOFFYear_YEAR] -> bus_creator/23
  [VINP_ReserveChargeOnDay_DAY] -> bus_creator/24
  [VINP_ReserveChargeOnHour_hr] -> bus_creator/25
  [VINP_ReserveChargeOnMinute_min] -> bus_creator/26
  [VINP_ReserveChargeOnMonth_MONTH] -> bus_creator/27
  [VINP_ReserveChargeOnYear_YEAR] -> bus_creator/28
  [VINP_TBOXHWVER_enum] -> bus_creator/29
  [VINP_TBOXSWVER_enum] -> bus_creator/30

== system inp/INP/CAN6/CommunicationCheck ==
  BHAL_outputs : Inport
  CANMsgInvalidFCM1 : FVT_lib/inp/CAN_Msg_Validity_Process_template  SystemSampleTime=-1  VariantActivationTime=update diagram  Latency=0  AutoFrameSizeCalculation=off
      link override ovrdflg: Value=KINP_CANMsgInvalidFCM1_flg_ovrdflg
      link override ovrdval: Value=KINP_CANMsgInvalidFCM1_flg_ovrdval
  CANMsgInvalidFCM3 : FVT_lib/inp/CAN_Msg_Validity_Process_template  SystemSampleTime=-1  VariantActivationTime=update diagram  Latency=0  AutoFrameSizeCalculation=off
      link override ovrdflg: Value=KINP_CANMsgInvalidFCM3_flg_ovrdflg
      link override ovrdval: Value=KINP_CANMsgInvalidFCM3_flg_ovrdval
  CANMsgInvalidSRR1 : FVT_lib/inp/CAN_Msg_Validity_Process_template  SystemSampleTime=-1  VariantActivationTime=update diagram  Latency=0  AutoFrameSizeCalculation=off
      link override ovrdflg: Value=KINP_CANMsgInvalidSRR1_flg_ovrdflg
      link override ovrdval: Value=KINP_CANMsgInvalidSRR1_flg_ovrdval
  bus_creator : BusCreator  Inputs=3
  bus_selector : BusSelector  OutputSignals=VHAL_CANMsgInvalidFCM1_flg,VHAL_CANMsgInvalidFCM3_flg,VHAL_CANMsgInvalidSRR1_flg
  not1 : Logic  Operator=NOT  AllPortsSameDT=off  OutDataTypeStr=boolean
  not2 : Logic  Operator=NOT  AllPortsSameDT=off  OutDataTypeStr=boolean
  not3 : Logic  Operator=NOT  AllPortsSameDT=off  OutDataTypeStr=boolean
  inp_CanValid_bus : Outport
  wires:
  BHAL_outputs/1 -> [BHAL_outputs]
  bus_selector/1 -> CANMsgInvalidFCM1/1  "<VHAL_CANMsgInvalidFCM1_flg>"
  CANMsgInvalidFCM1/1 -> not1/1
  not1/1 -> bus_creator/1  "VINP_CANMsgValidFCM1_flg"
  bus_selector/2 -> CANMsgInvalidFCM3/1  "<VHAL_CANMsgInvalidFCM3_flg>"
  CANMsgInvalidFCM3/1 -> not2/1
  not2/1 -> bus_creator/2  "VINP_CANMsgValidFCM3_flg"
  bus_selector/3 -> CANMsgInvalidSRR1/1  "<VHAL_CANMsgInvalidSRR1_flg>"
  CANMsgInvalidSRR1/1 -> not3/1
  not3/1 -> bus_creator/3  "VINP_CANMsgValidSRR1_flg"
  [BHAL_outputs] -> bus_selector/1
  bus_creator/1 -> inp_CanValid_bus/1
